simulink model "SimplifiedPowerPlantGeneratorToTransmissionGrid"  (R2022a)
settings: Solver=VariableStepAuto  StartTime=0.0  StopTime=5  RelTol=1e-3
undefined symbols (not defined in the file or in its folder): D1, Delta
libraries: spsSimplifiedSynchronousMachinepuUnitsLib x1, spsThreePhaseTransformerTwoWindingsLib x1, spsThreePhaseSourceLib x1, spspowerguiLib x1
settings Model: Creator=rodne  LastModifiedBy=rodne

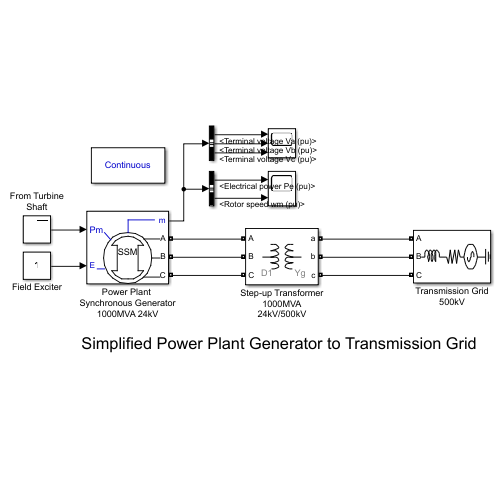
[thumbnail: Simulink's stored preview of the top-level diagram]
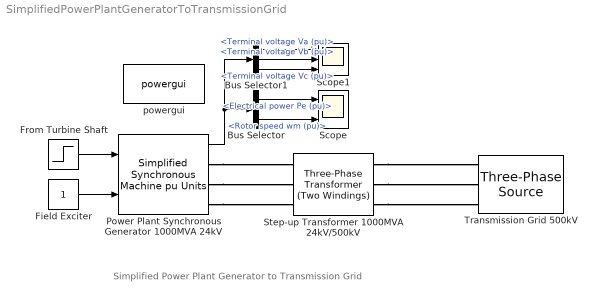
== system SimplifiedPowerPlantGeneratorToTransmissionGrid ==
  note: Simplified Power Plant Generator to Transmission Grid
  Bus Selector : BusSelector  OutputSignals=Electrical power Pe (pu),Rotor speed wm (pu)
  Bus Selector1 : BusSelector  OutputSignals=Terminal voltage Va (pu),Terminal voltage Vb (pu),Terminal voltage Vc (pu)
  Field Exciter : Constant
  From Turbine Shaft : Step  Time=2.5  Before=0.5  SampleTime=0
  Power Plant Synchronous Generator 1000MVA 24kV : spsSimplifiedSynchronousMachinepuUnitsLib/Simplified Synchronous Machine pu Units  ConnectionType=3-wire Y  MechanicalLoad=Mechanical power Pm  MeasurementBus=off  NominalParameters=[1000e6 24000 50]  Mechanical=[3.7 100 2]  InternalRL="[0.02  0.3]"  InitialConditions="[ 0,0   0,0,0   0,0,0 ]"  IterativeDiscreteModel=Trapezoidal non iterative  TsBlock=-1  TsPowergui=0  LoadFlowParameters=[1,0,0,0,0]  Units=0  BusType=PV  Pref=0  Qref=0  Qmin=-inf  Qmax=+inf  PLF=0  QLF=0
      settings: SourceProductBaseCode=PS
  Scope : Scope  NumInputPorts=2
  Scope1 : Scope  NumInputPorts=3
  Step-up Transformer 1000MVA 24kV/500kV : spsThreePhaseTransformerTwoWindingsLib/Three-Phase Transformer (Two Windings)  Winding1Connection=Delta (D1)  Winding2Connection=Yg  CoreType=Three single-phase transformers  SetSaturation=off  Hysteresis=off  DataFile='hysteresis'  SetInitialFlux=off  Measurements=None  UNITS=pu  NominalPower=[ 1000e6 , 50 ]  Winding1=[ 24e3 , 0.002 , 0 ]  Winding2=[ 500e3 , 0.002 , 0.08 ]  Rm=500  Lm=500  L0=0.5  Saturation=[ 0,0 ; 0.0024,1.2 ; 1.0,1.52 ]  InitialFluxes=[ 0.8 , -0.8 , 0.7 ]  BreakLoop=off  DiscreteSolver=Trapezoidal iterative  DataType=off  TransfoNumber=1
  Transmission Grid 500kV : spsThreePhaseSourceLib/Three-Phase Source  InternalConnection=Yg  VoltagePhases=off  Voltage=500e3  PhaseAngle=0  Voltage_phases=[25e3 25e3 25e3]/sqrt(3)  PhaseAngles_phases=[0 -120 +120]  Frequency=50  NonIdealSource=on  SpecifyImpedance=off  Resistance=0.8929  Inductance=16.58e-3  ShortCircuitLevel=100e6  BaseVoltage=500e3  XRratio=7  BusType=swing  Pref=10e3  Qref=0  Prefabc=[10e3, 10e3, 10e3]  Qrefabc=[0, 0, 0]  Qmin=-inf  Qmax=inf
  powergui : spspowerguiLib/powergui  Priority=1  SimulationMode=Continuous  SampleTime=50e-6  frequency=60  Iterations=50  frequencyindice=50  Pbase=100e6  ErrMax=1e-4  UnitsV=kV  UnitsW=MW  buscounter=0  FunctionMessages=off  echomessages=off  EnableUseOfTLC=off  CurrentSourceSwitches=off  DisableSnubberDevices=off  DisableRonSwitches=off  DisableVfSwitches=off  DisplayEquations=off  AutomaticDiscreteSolvers=off  SolverType=Tustin/Backward Euler (TBE)  Interpol=off  ExternalGateDelay=off  methode=off  Ts=100  x0status=blocks  SPID=on  SwTol=0  HookPort=off  NonlinearTolerance=1e-4  nMaxIteration=100  ContinueOnMaxIteration=off  RestoreLinks=warning  ResistiveCurrentMeasurement=off  Frange=[0:2:500]  Ylog=off  Xlog=on  ShowGrid=off  save=off  variable=ZData  structure=0  ZoomFFT=off  StartTime=0.0  cycles=1  DisplayStyle=1  fundamental=60  FreqAxis=off  MaxFrequency=1000  frequencyindicesteady=1  RmsSteady=1  display=off
  wires:
  Power Plant Synchronous Generator 1000MVA 24kV/1 -> Bus Selector1/1, Bus Selector/1
  Field Exciter/1 -> Power Plant Synchronous Generator 1000MVA 24kV/2
  Bus Selector/1 -> Scope/1  "<Electrical power Pe (pu)>"
  Bus Selector/2 -> Scope/2  "<Rotor speed wm (pu)>"
  From Turbine Shaft/1 -> Power Plant Synchronous Generator 1000MVA 24kV/1
  Bus Selector1/2 -> Scope1/2  "<Terminal voltage Vb (pu)>"
  Bus Selector1/1 -> Scope1/1  "<Terminal voltage Va (pu)>"
  Bus Selector1/3 -> Scope1/3  "<Terminal voltage Vc (pu)>"
  connections:
  Step-up Transformer 1000MVA 24kV/500kV/RConn2 -- Transmission Grid 500kV/RConn2
  Step-up Transformer 1000MVA 24kV/500kV/RConn1 -- Transmission Grid 500kV/RConn1
  Step-up Transformer 1000MVA 24kV/500kV/RConn3 -- Transmission Grid 500kV/RConn3
  Power Plant Synchronous Generator 1000MVA 24kV/RConn2 -- Step-up Transformer 1000MVA 24kV/500kV/LConn2
  Power Plant Synchronous Generator 1000MVA 24kV/RConn1 -- Step-up Transformer 1000MVA 24kV/500kV/LConn1
  Power Plant Synchronous Generator 1000MVA 24kV/RConn3 -- Step-up Transformer 1000MVA 24kV/500kV/LConn3
